simulink model "clic"  (R2017a)
settings: Solver=VariableStepAuto  StartTime=0.0  StopTime=6  RelTol=1e-3
libraries: simulink x18, dspinverses x1, sharedtransform x1, UR3_Lib x1, anthro_Lib x1
settings Model: Creator=dscat  LastModifiedBy=dscat

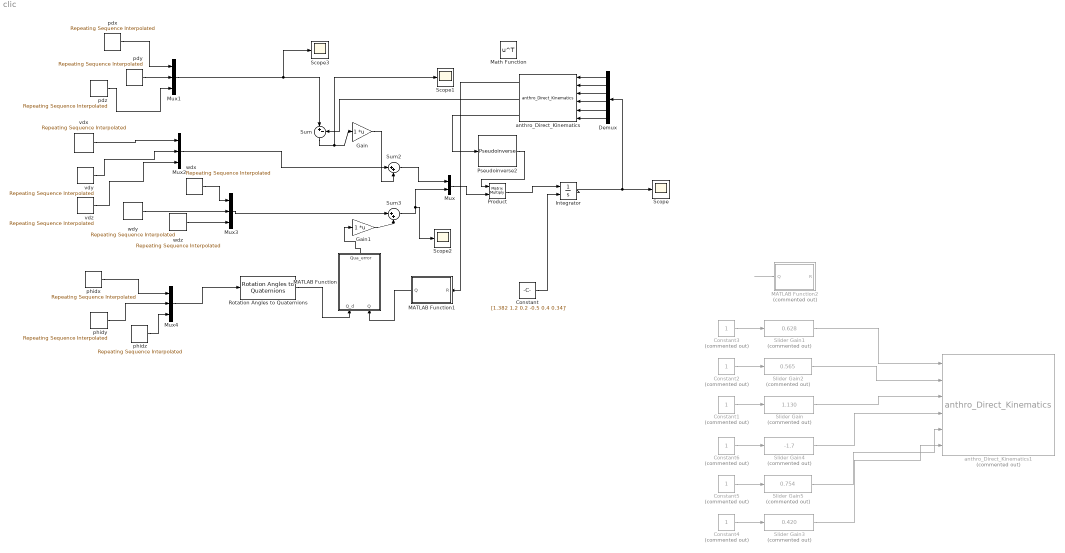
== system clic ==
  Constant : Constant  Value=[1.382 1.2 0.2 -0.5 0.4 0.34]'
  Constant{1..6} (6 alike) : Constant  Commented=on
  Demux : Demux  Outputs=6
  Gain : Gain  Multiplication=Matrix(K*u)
  Gain1 : Gain  Multiplication=Matrix(K*u)
  Integrator : Integrator  InitialConditionSource=external
  MATLAB Function : MATLAB Function  TreatAsAtomicUnit=on
  MATLAB Function1 : MATLAB Function  TreatAsAtomicUnit=on
  MATLAB Function2 : MATLAB Function  Commented=on  TreatAsAtomicUnit=on
  Math Function : Math  Operator=transpose  SaturateOnIntegerOverflow=on
  Mux : Mux  Inputs=2
  Mux{1..4} (4 alike) : Mux  Inputs=3
  Product : Product  Multiplication=Matrix(*)
  Pseudoinverse2 : dspinverses/Pseudoinverse  wanterr=off  SimulateUsing=Interpreted execution
      settings: SourceProductName=DSP System Toolbox  SourceProductBaseCode=DS
  Rotation Angles to Quaternions : sharedtransform/Rotation Angles to Quaternions  rotationOrder=ZYX
  Scope{,1..3} (4 alike) : Scope
  Slider Gain : simulink/Math Operations/Slider Gain  Commented=on  gain=1.130  low=-3.14  high=3.14
  Slider Gain1 : simulink/Math Operations/Slider Gain  Commented=on  gain=0.628  low=-3.14  high=3.14
  Slider Gain2 : simulink/Math Operations/Slider Gain  Commented=on  gain=0.565  low=-3.14  high=3.14
  Slider Gain3 : simulink/Math Operations/Slider Gain  Commented=on  gain=0.420  low=-1  high=1
  Slider Gain4 : simulink/Math Operations/Slider Gain  Commented=on  gain=-1.7  low=-3.14  high=3.14
  Slider Gain5 : simulink/Math Operations/Slider Gain  Commented=on  gain=0.754  low=-3.14  high=3.14
  Sum : Sum  Inputs=|+-
  Sum2 : Sum  Inputs=|++
  Sum3 : Sum  Inputs=|++
  anthro_Direct_Kinematics : UR3_Lib/anthro_Direct_Kinematics
  anthro_Direct_Kinematics1 : anthro_Lib/anthro_Direct_Kinematics  Commented=on
  pdx : simulink/Sources/Repeating Sequence Interpolated  OutValues=pdx  TimeValues=t  LookUpMeth=Interpolation-Use End Values  tsamp=0.01  OutMin=[]  OutMax=[]  OutDataTypeStr=double  OutputDataTypeScalingMode=double  OutDataType=fixdt(0,8)  OutScaling=2^-10
  pdy : simulink/Sources/Repeating Sequence Interpolated  OutValues=pdy  TimeValues=t  LookUpMeth=Interpolation-Use End Values  tsamp=0.01  OutMin=[]  OutMax=[]  OutDataTypeStr=double  OutputDataTypeScalingMode=double  OutDataType=fixdt(0,8)  OutScaling=2^-10
  pdz : simulink/Sources/Repeating Sequence Interpolated  OutValues=pdz  TimeValues=t  LookUpMeth=Interpolation-Use End Values  tsamp=0.01  OutMin=[]  OutMax=[]  OutDataTypeStr=double  OutputDataTypeScalingMode=double  OutDataType=fixdt(0,8)  OutScaling=2^-10
  phidx : simulink/Sources/Repeating Sequence Interpolated  OutValues=phidx  TimeValues=t  LookUpMeth=Interpolation-Use End Values  tsamp=0.01  OutMin=[]  OutMax=[]  OutDataTypeStr=double  OutputDataTypeScalingMode=double  OutDataType=fixdt(0,8)  OutScaling=2^-10
  phidy : simulink/Sources/Repeating Sequence Interpolated  OutValues=phidy  TimeValues=t  LookUpMeth=Interpolation-Use End Values  tsamp=0.01  OutMin=[]  OutMax=[]  OutDataTypeStr=double  OutputDataTypeScalingMode=double  OutDataType=fixdt(0,8)  OutScaling=2^-10
  phidz : simulink/Sources/Repeating Sequence Interpolated  OutValues=phidz  TimeValues=t  LookUpMeth=Interpolation-Use End Values  tsamp=0.01  OutMin=[]  OutMax=[]  OutDataTypeStr=double  OutputDataTypeScalingMode=double  OutDataType=fixdt(0,8)  OutScaling=2^-10
  vdx : simulink/Sources/Repeating Sequence Interpolated  OutValues=vdx  TimeValues=t  LookUpMeth=Interpolation-Use End Values  tsamp=0.01  OutMin=[]  OutMax=[]  OutDataTypeStr=double  OutputDataTypeScalingMode=double  OutDataType=fixdt(0,8)  OutScaling=2^-10
  vdy : simulink/Sources/Repeating Sequence Interpolated  OutValues=vdy  TimeValues=t  LookUpMeth=Interpolation-Use End Values  tsamp=0.01  OutMin=[]  OutMax=[]  OutDataTypeStr=double  OutputDataTypeScalingMode=double  OutDataType=fixdt(0,8)  OutScaling=2^-10
  vdz : simulink/Sources/Repeating Sequence Interpolated  OutValues=vdz  TimeValues=t  LookUpMeth=Interpolation-Use End Values  tsamp=0.01  OutMin=[]  OutMax=[]  OutDataTypeStr=double  OutputDataTypeScalingMode=double  OutDataType=fixdt(0,8)  OutScaling=2^-10
  "wdx " : simulink/Sources/Repeating Sequence Interpolated  OutValues=wdx  TimeValues=t  LookUpMeth=Interpolation-Use End Values  tsamp=0.01  OutMin=[]  OutMax=[]  OutDataTypeStr=double  OutputDataTypeScalingMode=double  OutDataType=fixdt(0,8)  OutScaling=2^-10
  wdy : simulink/Sources/Repeating Sequence Interpolated  OutValues=wdy  TimeValues=t  LookUpMeth=Interpolation-Use End Values  tsamp=0.01  OutMin=[]  OutMax=[]  OutDataTypeStr=double  OutputDataTypeScalingMode=double  OutDataType=fixdt(0,8)  OutScaling=2^-10
  wdz : simulink/Sources/Repeating Sequence Interpolated  OutValues=wdz  TimeValues=t  LookUpMeth=Interpolation-Use End Values  tsamp=0.01  OutMin=[]  OutMax=[]  OutDataTypeStr=double  OutputDataTypeScalingMode=double  OutDataType=fixdt(0,8)  OutScaling=2^-10
  wires:
  Sum/1 -> Scope1/1, Gain/1
  Gain/1 -> Sum2/2
  Sum2/1 -> Mux/1
  MATLAB Function/1(Qua_error) -> Gain1/1
  Gain1/1 -> Sum3/2
  Sum3/1 -> Scope2/1, Mux/2
  anthro_Direct_Kinematics/3 -> Pseudoinverse2/1
  anthro_Direct_Kinematics/1 -> MATLAB Function1/1(R)
  Rotation Angles to Quaternions/1 -> MATLAB Function/1(Q_d)
  MATLAB Function1/1(Q) -> MATLAB Function/2(Q)
  Product/1 -> Integrator/1
  Mux/1 -> Product/2
  Demux/5 -> anthro_Direct_Kinematics/5
  Integrator/1 -> Scope/1, Demux/1
  anthro_Direct_Kinematics/2 -> Sum/2
  Constant/1 -> Integrator/2
  vdx/1 -> Mux2/1
  Mux1/1 -> Scope3/1, Sum/1
  vdy/1 -> Mux2/2
  vdz/1 -> Mux2/3
  Mux2/1 -> Sum2/1
  Mux3/1 -> Sum3/1
  Mux4/1 -> Rotation Angles to Quaternions/1
  Constant6/1 -> Slider Gain4/1
  Constant3/1 -> Slider Gain1/1
  Constant4/1 -> Slider Gain3/1
  Constant2/1 -> Slider Gain2/1
  Slider Gain5/1 -> anthro_Direct_Kinematics1/5
  Slider Gain2/1 -> anthro_Direct_Kinematics1/2
  Slider Gain3/1 -> anthro_Direct_Kinematics1/6
  Slider Gain4/1 -> anthro_Direct_Kinematics1/4
  Constant5/1 -> Slider Gain5/1
  Slider Gain/1 -> anthro_Direct_Kinematics1/3
  Slider Gain1/1 -> anthro_Direct_Kinematics1/1
  Constant1/1 -> Slider Gain/1
  MATLAB Function2/1(Q) -> ?
  pdx/1 -> Mux1/1
  pdy/1 -> Mux1/2
  pdz/1 -> Mux1/3
  "wdx "/1 -> Mux3/1
  wdy/1 -> Mux3/2
  wdz/1 -> Mux3/3
  phidz/1 -> Mux4/3
  phidy/1 -> Mux4/2
  phidx/1 -> Mux4/1
  Pseudoinverse2/1 -> Product/1
  Demux/6 -> anthro_Direct_Kinematics/6
  Demux/3 -> anthro_Direct_Kinematics/3
  Demux/1 -> anthro_Direct_Kinematics/1
  Demux/4 -> anthro_Direct_Kinematics/4
  Demux/2 -> anthro_Direct_Kinematics/2

== matlab function clic/MATLAB Function1 ==
  data: R input; Q output
function Q   = Rot_Quar( R )
%This function converts the rotation matrix into Quarternion Representation
Q=zeros(4,1);

etta=1/2*sqrt(abs(R(1,1)+R(2,2)+R(3,3)+1));
epsilon1=1/2*sign(R(3,2)-R(2,3))*sqrt(abs(R(1,1)-R(2,2)-R(3,3)+1));
epsilon2=1/2*sign(R(1,3)-R(3,1))*sqrt(abs(R(2,2)-R(3,3)-R(1,1)+1));
epsilon3=1/2*sign(R(2,1)-R(1,2))*sqrt(abs(R(3,3)-R(1,1)-R(2,2)+1));

Q=[etta;epsilon1;epsilon2;epsilon3];
end

== matlab function clic/MATLAB Function ==
  data: Q_d input; Qua_error output; Q input
function Qua_error   = error_Q( Q_d, Q )
%This function computes the error of the current quarternion configuration
Qua_error=zeros(3,1);
Qua_error=Q(1)*Q_d(2:4)-Q_d(1)*Q(2:4)-cross(Q_d(2:4),Q(2:4));

end

== matlab function clic/MATLAB Function2 ==
  data: R input; Q output
function Q   = Rot_Quar( R )
%This function converts the rotation matrix into Quarternion Representation
Q=zeros(4,1);

etta=1/2*sqrt(abs(R(1,1)+R(2,2)+R(3,3)+1));
epsilon1=1/2*sign(R(3,2)-R(2,3))*sqrt(abs(R(1,1)-R(2,2)-R(3,3)+1));
epsilon2=1/2*sign(R(1,3)-R(3,1))*sqrt(abs(R(2,2)-R(3,3)-R(1,1)+1));
epsilon3=1/2*sign(R(2,1)-R(1,2))*sqrt(abs(R(3,3)-R(1,1)-R(2,2)+1));

Q=[etta;epsilon1;epsilon2;epsilon3];
end
